simulink model "open_differential_no_PID"  (R2024b)
settings: Solver=VariableStepAuto  StartTime=0.0  StopTime=10.0  RelTol=1e-3
libraries: simulink x4
settings Model: Creator=chris  LastModifiedBy=chris

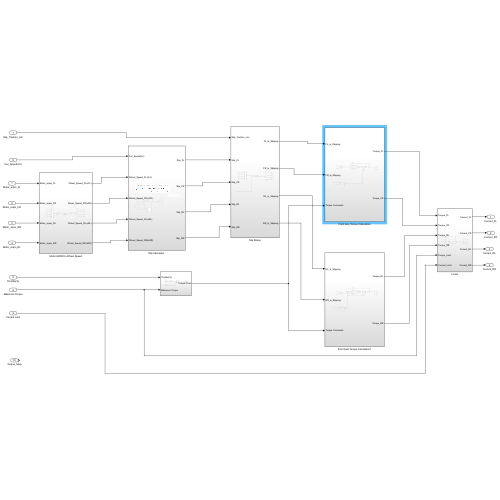
[thumbnail: Simulink's stored preview of the top-level diagram]
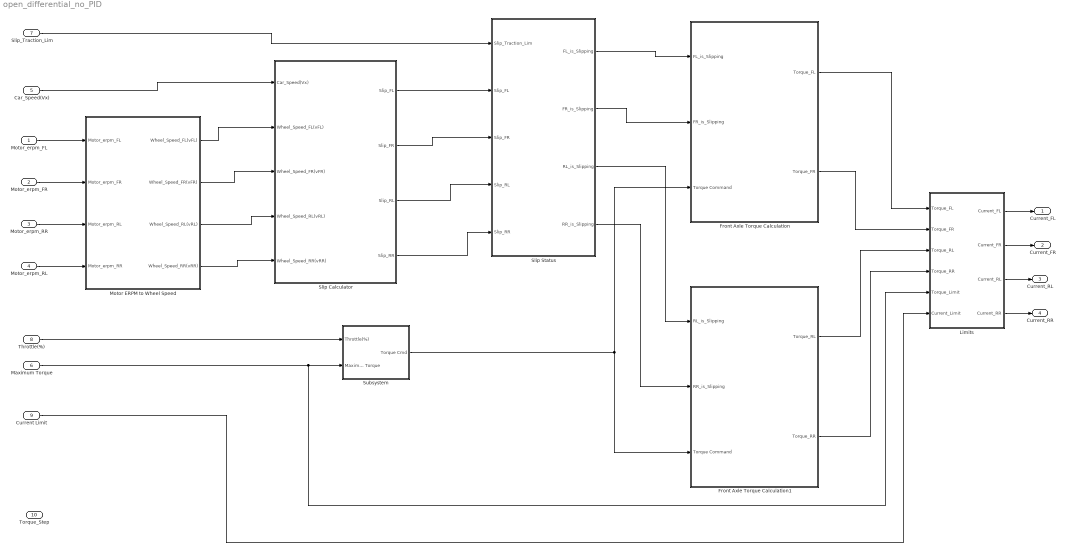
== system open_differential_no_PID ==
  Motor_erpm_FL : Inport
  Motor_erpm_FR : Inport  Port=2
  Motor_erpm_RR : Inport  Port=3
  Motor_erpm_RL : Inport  Port=4
  Car_Speed(Vx) : Inport  Port=5
  Maximum Torque : Inport  Port=6
  Slip_Traction_Lim : Inport  Port=7
  Throttle(%) : Inport  Port=8
  Current Limit : Inport  Port=9
  Torque_Step : Inport  Port=10
  Front Axle Torque Calculation : Subsystem
  Front Axle Torque Calculation1 : Subsystem
  Limits : Subsystem
  Motor ERPM to Wheel Speed : Subsystem
  "Slip Calculator " : Subsystem
  Slip Status : Subsystem
  Subsystem : Subsystem
  Current_FL : Outport
  Current_FR : Outport  Port=2
  Current_RL : Outport  Port=3
  Current_RR : Outport  Port=4
  wires:
  Slip_Traction_Lim/1 -> Slip Status/1(Slip_Traction_Lim)
  Front Axle Torque Calculation/1(Torque_FL) -> Limits/1(Torque_FL)
  Current Limit/1 -> Limits/6(Current_Limit)
  Throttle(%)/1 -> Subsystem/1(Throttle(%))
  Maximum Torque/1 -> Limits/5(Torque_Limit), Subsystem/2(Maximum Torque)
  "Slip Calculator "/1(Slip_FL) -> Slip Status/2(Slip_FL)
  "Slip Calculator "/4(Slip_RR) -> Slip Status/5(Slip_RR)
  Limits/2(Current_FR) -> Current_FR/1
  Limits/4(Current_RR) -> Current_RR/1
  Limits/1(Current_FL) -> Current_FL/1
  Limits/3(Current_RL) -> Current_RL/1
  "Slip Calculator "/2(Slip_FR) -> Slip Status/3(Slip_FR)
  "Slip Calculator "/3(Slip_RL) -> Slip Status/4(Slip_RL)
  Front Axle Torque Calculation/2(Torque_FR) -> Limits/2(Torque_FR)
  Subsystem/1(Torque Cmd) -> Front Axle Torque Calculation/3(Torque Command), Front Axle Torque Calculation1/3(Torque Command)
  Car_Speed(Vx)/1 -> "Slip Calculator "/1(Car_Speed(Vx))
  Motor_erpm_FL/1 -> Motor ERPM to Wheel Speed/1(Motor_erpm_FL)
  Motor_erpm_FR/1 -> Motor ERPM to Wheel Speed/2(Motor_erpm_FR)
  Motor_erpm_RR/1 -> Motor ERPM to Wheel Speed/3(Motor_erpm_RL)
  Motor_erpm_RL/1 -> Motor ERPM to Wheel Speed/4(Motor_erpm_RR)
  Motor ERPM to Wheel Speed/1(Wheel_Speed_FL(vFL)) -> "Slip Calculator "/2(Wheel_Speed_FL(vFL))
  Motor ERPM to Wheel Speed/2(Wheel_Speed_FR(vFR)) -> "Slip Calculator "/3(Wheel_Speed_FR(vFR))
  Motor ERPM to Wheel Speed/3(Wheel_Speed_RL(vRL)) -> "Slip Calculator "/4(Wheel_Speed_RL(vRL))
  Motor ERPM to Wheel Speed/4(Wheel_Speed_RR(vRR)) -> "Slip Calculator "/5(Wheel_Speed_RR(vRR))
  Slip Status/1(FL_is_Slipping) -> Front Axle Torque Calculation/1(FL_is_Slipping)
  Slip Status/2(FR_is_Slipping) -> Front Axle Torque Calculation/2(FR_is_Slipping)
  Slip Status/3(RL_is_Slipping) -> Front Axle Torque Calculation1/1(RL_is_Slipping)
  Slip Status/4(RR_is_Slipping) -> Front Axle Torque Calculation1/2(RR_is_Slipping)
  Front Axle Torque Calculation1/1(Torque_RL) -> Limits/3(Torque_RL)
  Front Axle Torque Calculation1/2(Torque_RR) -> Limits/4(Torque_RR)

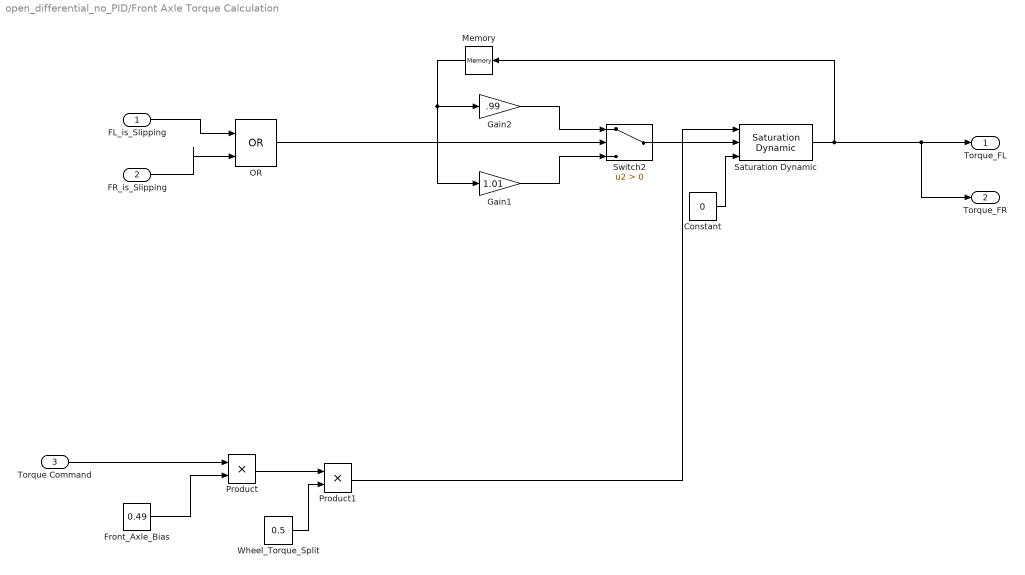
== system open_differential_no_PID/Front Axle Torque Calculation ==
  FL_is_Slipping : Inport
  FR_is_Slipping : Inport  Port=2
  Torque Command : Inport  Port=3
  Constant : Constant  Value=0
  Front_Axle_Bias : Constant  Value=0.49
  Gain1 : Gain  Gain=1.01
  Gain2 : Gain  Gain=.99
  Memory : Memory  InitialCondition=1
  OR : Logic  Operator=OR  IconShape=distinctive  AllPortsSameDT=off  OutDataTypeStr=boolean
  Product : Product
  Product1 : Product
  Saturation Dynamic : simulink/Discontinuities/Saturation Dynamic  OutMin=[]  OutMax=[]  OutDataTypeStr=Inherit: Same as second input  OutDataType=fixdt(1, 16)  OutScaling=2^-10  DoSatur=off
  Switch2 : Switch  Criteria=u2 > Threshold  SaturateOnIntegerOverflow=off  InputSameDT=off
  Wheel_Torque_Split : Constant  Value=0.5
  Torque_FL : Outport
  Torque_FR : Outport  Port=2
  wires:
  Torque Command/1 -> Product/1
  Front_Axle_Bias/1 -> Product/2
  Product/1 -> Product1/1
  Wheel_Torque_Split/1 -> Product1/2
  FL_is_Slipping/1 -> OR/1
  FR_is_Slipping/1 -> OR/2
  OR/1 -> Switch2/2
  Memory/1 -> Gain2/1, Gain1/1
  Gain1/1 -> Switch2/3
  Switch2/1 -> Saturation Dynamic/2
  Constant/1 -> Saturation Dynamic/3
  Gain2/1 -> Switch2/1
  Saturation Dynamic/1 -> Memory/1, Torque_FR/1, Torque_FL/1
  Product1/1 -> Saturation Dynamic/1

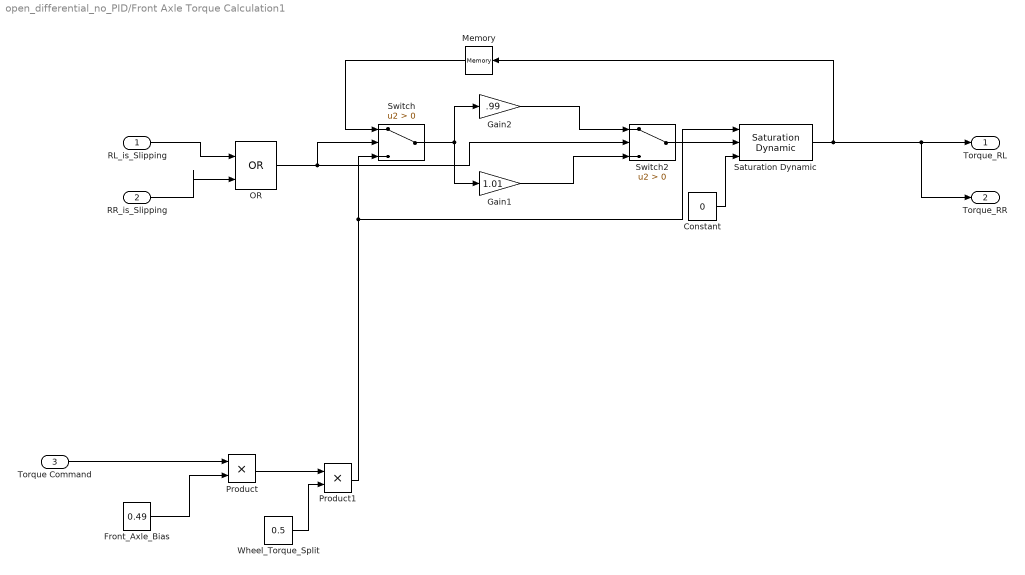
== system open_differential_no_PID/Front Axle Torque Calculation1 ==
  RL_is_Slipping : Inport
  RR_is_Slipping : Inport  Port=2
  Torque Command : Inport  Port=3
  Constant : Constant  Value=0
  Front_Axle_Bias : Constant  Value=0.49
  Gain1 : Gain  Gain=1.01
  Gain2 : Gain  Gain=.99
  Memory : Memory
  OR : Logic  Operator=OR  IconShape=distinctive  AllPortsSameDT=off  OutDataTypeStr=boolean
  Product : Product
  Product1 : Product
  Saturation Dynamic : simulink/Discontinuities/Saturation Dynamic  OutMin=[]  OutMax=[]  OutDataTypeStr=Inherit: Same as second input  OutDataType=fixdt(1, 16)  OutScaling=2^-10  DoSatur=off
  Switch : Switch  Criteria=u2 > Threshold  SaturateOnIntegerOverflow=off  InputSameDT=off
  Switch2 : Switch  Criteria=u2 > Threshold  SaturateOnIntegerOverflow=off  InputSameDT=off
  Wheel_Torque_Split : Constant  Value=0.5
  Torque_RL : Outport
  Torque_RR : Outport  Port=2
  wires:
  Torque Command/1 -> Product/1
  Front_Axle_Bias/1 -> Product/2
  Product/1 -> Product1/1
  Wheel_Torque_Split/1 -> Product1/2
  Memory/1 -> Switch/1
  Product1/1 -> Saturation Dynamic/1, Switch/3
  RL_is_Slipping/1 -> OR/1
  RR_is_Slipping/1 -> OR/2
  OR/1 -> Switch2/2, Switch/2
  Switch/1 -> Gain2/1, Gain1/1
  Gain1/1 -> Switch2/3
  Switch2/1 -> Saturation Dynamic/2
  Constant/1 -> Saturation Dynamic/3
  Gain2/1 -> Switch2/1
  Saturation Dynamic/1 -> Memory/1, Torque_RR/1, Torque_RL/1

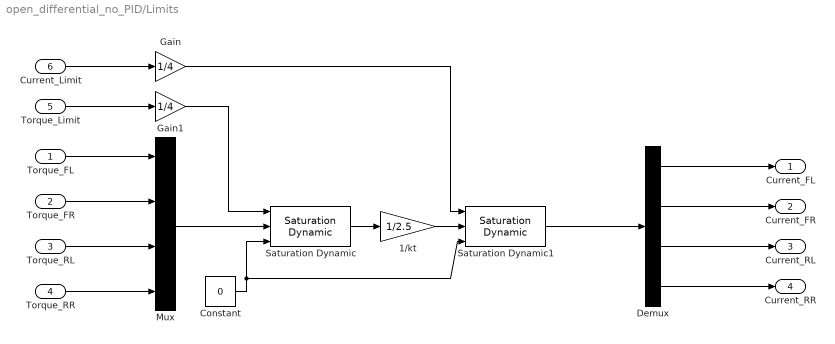
== system open_differential_no_PID/Limits ==
  Torque_FL : Inport
  Torque_FR : Inport  Port=2
  Torque_RL : Inport  Port=3
  Torque_RR : Inport  Port=4
  Torque_Limit : Inport  Port=5
  Current_Limit : Inport  Port=6
  1/kt : Gain  Gain=1/2.5
  Constant : Constant  Value=0
  Demux : Demux
  Gain : Gain  Gain=1/4
  Gain1 : Gain  Gain=1/4
  Mux : Mux
  Saturation Dynamic : simulink/Discontinuities/Saturation Dynamic  OutMin=[]  OutMax=[]  OutDataTypeStr=Inherit: Same as second input  OutDataType=fixdt(1, 16)  OutScaling=2^-10  DoSatur=off
  Saturation Dynamic1 : simulink/Discontinuities/Saturation Dynamic  OutMin=[]  OutMax=[]  OutDataTypeStr=Inherit: Same as second input  OutDataType=fixdt(1, 16)  OutScaling=2^-10  DoSatur=off
  Current_FL : Outport
  Current_FR : Outport  Port=2
  Current_RL : Outport  Port=3
  Current_RR : Outport  Port=4
  wires:
  Torque_FR/1 -> Mux/2
  Torque_FL/1 -> Mux/1
  Torque_RL/1 -> Mux/3
  Torque_RR/1 -> Mux/4
  Mux/1 -> Saturation Dynamic/2
  Constant/1 -> Saturation Dynamic/3, Saturation Dynamic1/3
  Demux/1 -> Current_FL/1
  Demux/2 -> Current_FR/1
  Demux/3 -> Current_RL/1
  Demux/4 -> Current_RR/1
  Saturation Dynamic/1 -> 1/kt/1
  1/kt/1 -> Saturation Dynamic1/2
  Saturation Dynamic1/1 -> Demux/1
  Torque_Limit/1 -> Gain1/1
  Current_Limit/1 -> Gain/1
  Gain/1 -> Saturation Dynamic1/1
  Gain1/1 -> Saturation Dynamic/1

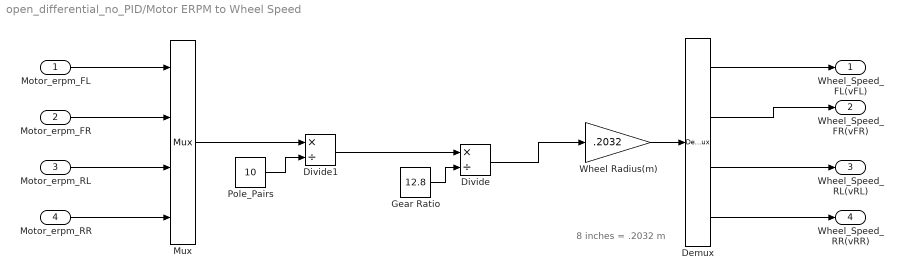
== system open_differential_no_PID/Motor ERPM to Wheel Speed ==
  note: 8 inches = .2032 m
  Motor_erpm_FL : Inport
  Motor_erpm_FR : Inport  Port=2
  Motor_erpm_RL : Inport  Port=3
  Motor_erpm_RR : Inport  Port=4
  Demux : Demux
  Divide : Product  Inputs=*/
  Divide1 : Product  Inputs=*/
  Gear Ratio : Constant  Value=12.8
  Mux : Mux
  Pole_Pairs : Constant  Value=10
  Wheel Radius(m) : Gain  Gain=.2032
  Wheel_Speed_FL(vFL) : Outport
  Wheel_Speed_FR(vFR) : Outport  Port=2
  Wheel_Speed_RL(vRL) : Outport  Port=3
  Wheel_Speed_RR(vRR) : Outport  Port=4
  wires:
  Motor_erpm_FL/1 -> Mux/1
  Motor_erpm_FR/1 -> Mux/2
  Motor_erpm_RL/1 -> Mux/3
  Motor_erpm_RR/1 -> Mux/4
  Gear Ratio/1 -> Divide/2
  Divide/1 -> Wheel Radius(m)/1
  Mux/1 -> Divide1/1
  Pole_Pairs/1 -> Divide1/2
  Divide1/1 -> Divide/1
  Demux/1 -> Wheel_Speed_FL(vFL)/1
  Demux/2 -> Wheel_Speed_FR(vFR)/1
  Demux/3 -> Wheel_Speed_RL(vRL)/1
  Wheel Radius(m)/1 -> Demux/1
  Demux/4 -> Wheel_Speed_RR(vRR)/1

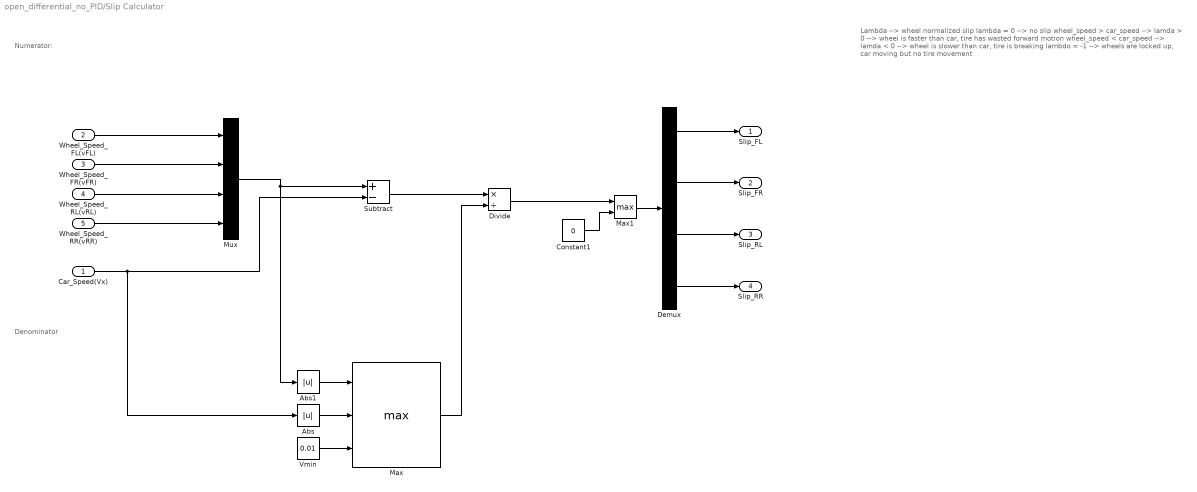
== system open_differential_no_PID/Slip Calculator  ==
  note: Lambda --> wheel normalized slip
      | lambda = 0 --> no slip
      | wheel_speed > car_speed --> lamda > 0 --> wheel is faster than car, tire has wasted forward motion
      | wheel_speed < car_speed --> lamda < 0 --> wheel is slower than car, tire is breaking
      | lambdo = -1 --> wheels are locked up, car moving but no tire movement
  note: Numerator:
  note: Denominator
  Car_Speed(Vx) : Inport
  Wheel_Speed_FL(vFL) : Inport  Port=2
  Wheel_Speed_FR(vFR) : Inport  Port=3
  Wheel_Speed_RL(vRL) : Inport  Port=4
  Wheel_Speed_RR(vRR) : Inport  Port=5
  Abs : Abs  SaturateOnIntegerOverflow=off
  Abs1 : Abs  SaturateOnIntegerOverflow=off
  Constant1 : Constant  Value=0
  Demux : Demux
  Divide : Product  Inputs=*/
  Max : MinMax  Function=max  Inputs=3
  Max1 : MinMax  Function=max  Inputs=2
  Mux : Mux
  Subtract : Sum  Inputs=+-
  Vmin : Constant  Value=0.01
  Slip_FL : Outport
  Slip_FR : Outport  Port=2
  Slip_RL : Outport  Port=3
  Slip_RR : Outport  Port=4
  wires:
  Wheel_Speed_FL(vFL)/1 -> Mux/1
  Wheel_Speed_FR(vFR)/1 -> Mux/2
  Wheel_Speed_RL(vRL)/1 -> Mux/3
  Wheel_Speed_RR(vRR)/1 -> Mux/4
  Subtract/1 -> Divide/1
  Max/1 -> Divide/2
  Mux/1 -> Abs1/1, Subtract/1
  Constant1/1 -> Max1/2
  Max1/1 -> Demux/1
  Demux/4 -> Slip_RR/1
  Demux/3 -> Slip_RL/1
  Demux/2 -> Slip_FR/1
  Demux/1 -> Slip_FL/1
  Divide/1 -> Max1/1
  Vmin/1 -> Max/3
  Abs/1 -> Max/2
  Car_Speed(Vx)/1 -> Abs/1, Subtract/2
  Abs1/1 -> Max/1

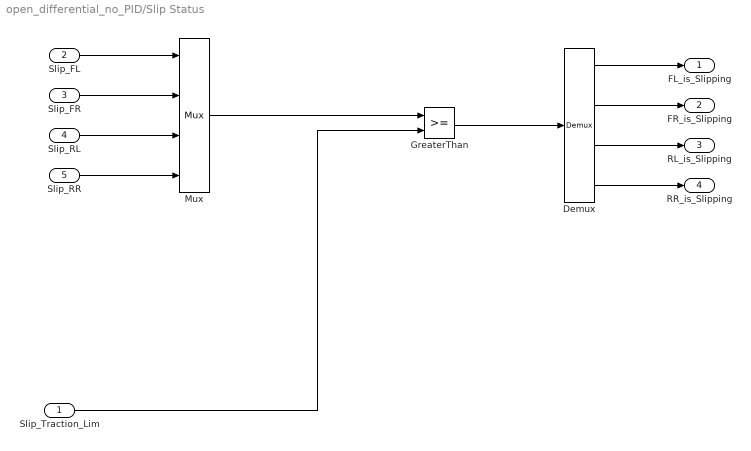
== system open_differential_no_PID/Slip Status ==
  Slip_Traction_Lim : Inport
  Slip_FL : Inport  Port=2
  Slip_FR : Inport  Port=3
  Slip_RL : Inport  Port=4
  Slip_RR : Inport  Port=5
  Demux : Demux
  GreaterThan : RelationalOperator  OutDataTypeStr=boolean  RndMeth=Simplest  InputSameDT=off
  Mux : Mux
  FL_is_Slipping : Outport
  FR_is_Slipping : Outport  Port=2
  RL_is_Slipping : Outport  Port=3
  RR_is_Slipping : Outport  Port=4
  wires:
  Slip_RR/1 -> Mux/4
  Slip_RL/1 -> Mux/3
  Slip_FR/1 -> Mux/2
  Slip_FL/1 -> Mux/1
  Mux/1 -> GreaterThan/1
  Slip_Traction_Lim/1 -> GreaterThan/2
  GreaterThan/1 -> Demux/1
  Demux/1 -> FL_is_Slipping/1
  Demux/2 -> FR_is_Slipping/1
  Demux/4 -> RR_is_Slipping/1
  Demux/3 -> RL_is_Slipping/1

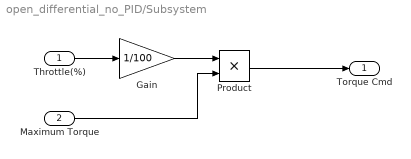
== system open_differential_no_PID/Subsystem ==
  Throttle(%) : Inport
  Maximum Torque : Inport  Port=2
  Gain : Gain  Gain=1/100
  Product : Product
  Torque Cmd : Outport
  wires:
  Throttle(%)/1 -> Gain/1
  Maximum Torque/1 -> Product/2
  Gain/1 -> Product/1
  Product/1 -> Torque Cmd/1
